simulink model "IARC_Nonlinear_Sensors"  (R2018a)
settings: Solver=ode1  StartTime=0.0  StopTime=20  FixedStep=T  RelTol=1e-3  EnableMultiTasking=on
undefined symbols (not defined in the file): A_1df, A_2df, alpha3, alpha_rp, alpha_x, alpha_z, an1, an1_v, an2, an3, bn1, bn1_v, bn2, bn3, dc_M_x, delta3, Epsilon3, F, g, Gamma1, Gamma2, Gamma3, Gamma4, gamma4_0, gamma_d_x, gamma_rp_0, gamma_x_0, gamma_z_0, Gammax, I, I_add, I_add_time, Jx, Jy, Jyaw, K, k1, k10, k11, k12, k2, k3, k4, k5, k6, k7, k8, k9, Ky, L, Light, LIMIT_CMD_PITCH, LIMIT_CMD_ROLL, LIMIT_CMD_xy, LIMIT_uCMD_HEIGHT, m, m_add, m_add_time, magnitude, MIL ... (+67)
libraries: simulink x131, simulink_extras x5, UAV_Control x4, aerolibwind2 x1
(part 2 of 6)

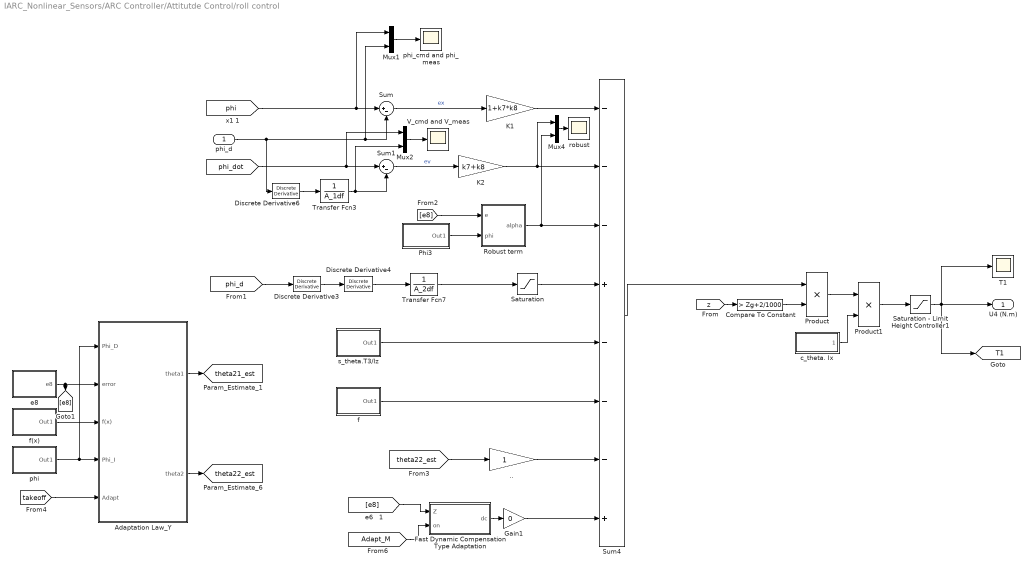
== system IARC_Nonlinear_Sensors/ARC Controller/Attitutde Control/roll control ==
  phi_d : Inport
  .. : Gain
  Adaptation Law_Y : Subsystem
  Compare To Constant : simulink/Logic and Bit Operations/Compare To Constant  relop=>  const=Zg+2/1000  OutDataTypeStr=uint8  ZeroCross=off
  Discrete Derivative3 : simulink/Discrete/Discrete Derivative  gainval=1.0  ICPrevScaledInput=0.0  OutMin=[]  OutMax=[]  OutDataType=fixdt(1, 16)  OutScaling=2^-10  DoSatur=off
  Discrete Derivative4 : simulink/Discrete/Discrete Derivative  gainval=1.0  ICPrevScaledInput=0.0  OutMin=[]  OutMax=[]  OutDataType=fixdt(1, 16)  OutScaling=2^-10  DoSatur=off
  Discrete Derivative6 : simulink/Discrete/Discrete Derivative  gainval=1.0  ICPrevScaledInput=0.0  OutMin=[]  OutMax=[]  OutDataType=fixdt(1, 16)  OutScaling=2^-10  DoSatur=off
  Fast Dynamic Compensation Type Adaptation : Subsystem  mask{dc_M=dc_M_x, gamma_d=gamma_d_x}
      mask prompts: dc_M "Bound for the lumped model compensation errors"; gamma_d "Adaptation gain:"
      mask Help:
      | d ̂  ̇_c=Proj(γ_d z)=0             if      |d ̂_c |=d_cM  and d ̂_c z>0
      |                                 γ_d z      else
      | With γ_d>0 and |d ̂_c (0)|≤d_cM
      mask Display:
      | port_label('input',1,'e','texmode','on')
      | port_label('output',1,'d_c','texmode','on')
  Gain1 : Gain  Gain=0
  K1 : Gain  Gain=1+k7*k8
  K2 : Gain  Gain=k7+k8
  Mux1 : Mux  Inputs=2
  Mux2 : Mux  Inputs=2
  Mux4 : Mux  Inputs=2
  Phi3 : Subsystem
  Product : Product  Inputs=**
  Product1 : Product
  Robust term : Subsystem  mask(Robust_Block){theta_max=theta3_Max, theta_min=theta3_Min, epsilon=Epsilon3, delta=delta3}
      mask prompts: theta_max "Maximum parameters vector value:"; theta_min "Minimum parameters vector value:"; epsilon "Error bound Coefficient:"; delta "Uncertain Nonlinearities Bound:"
      mask help: Computes the nonlinear robust feedback.
      mask Help:
      | h^2=(theta_max-theta_min)^2*phi^2+delta^2
      | u = h/(4epsilon) )e/theta
      mask Display:
      | port_label('input',1,'e','texmode','on')
      | port_label('input',2,'\phi','texmode','on')
      | 
      | port_label('output',1,'u_{s2}','texmode','on')
  Saturation : Saturate  UpperLimit=[10]  LowerLimit=[-10]
  Saturation - Limit Height Controller1 : Saturate  UpperLimit=0.8  LowerLimit=-0.8
  Sum : Sum  Inputs=|+-
  Sum1 : Sum  Inputs=|+-
  Sum4 : Sum  Inputs=---+---+
  T1 : Scope
  Transfer Fcn3 : TransferFcn  Denominator=A_1df
  Transfer Fcn7 : TransferFcn  Denominator=A_2df
  V_cmd and V_meas : Scope
  c_theta. Ix : Subsystem
  e8 : Subsystem
  f : Subsystem
  f(x) : Subsystem
  phi : Subsystem
  phi_cmd and phi_meas : Scope
  robust : Scope
  s_theta.T3/Iz : Subsystem
  U4 (N.m) : Outport
  tag scope: T1=global, theta21_est=global, theta22_est=global
  wires:
  Mux1/1 -> phi_cmd and phi_meas/1
  Sum/1 -> K1/1  "ex"
  [phi] -> Mux1/1, Sum/1
  [z] -> Compare To Constant/1
  Compare To Constant/1 -> Product/2
  Sum4/1 -> Product/1
  [phi_d] -> Discrete Derivative3/1
  Discrete Derivative3/1 -> Discrete Derivative4/1
  K1/1 -> Sum4/1
  K2/1 -> Mux4/1, Sum4/2
  Discrete Derivative4/1 -> Transfer Fcn7/1
  phi/1(Out1) -> Adaptation Law_Y/1(Phi_D), Adaptation Law_Y/4(Phi_I)
  [takeoff] -> Adaptation Law_Y/5(Adapt)
  f(x)/1(Out1) -> Adaptation Law_Y/3(f(x))
  Discrete Derivative6/1 -> Transfer Fcn3/1
  [phi_dot] -> Mux2/1, Sum1/1
  Mux2/1 -> V_cmd and V_meas/1
  e8/1(e8) -> Adaptation Law_Y/2(error), [e8]
  Adaptation Law_Y/2(theta2) -> [theta22_est]
  Adaptation Law_Y/1(theta1) -> [theta21_est]
  ../1 -> Sum4/7
  Product/1 -> Product1/1
  Phi3/1(Out1) -> Robust term/2(phi)
  Sum1/1 -> K2/1  "ev"
  [e8] -> Robust term/1(e)
  Robust term/1(alpha) -> Mux4/2, Sum4/3
  Product1/1 -> Saturation - Limit Height Controller1/1
  phi_d/1 -> Discrete Derivative6/1, Mux1/2, Sum/2
  [theta22_est] -> ../1
  s_theta.T3/Iz/1(Out1) -> Sum4/5
  f/1(Out1) -> Sum4/6
  Transfer Fcn3/1 -> Sum1/2, Mux2/2
  Saturation/1 -> Sum4/4
  Transfer Fcn7/1 -> Saturation/1
  c_theta. Ix/1(" ") -> Product1/2
  Saturation - Limit Height Controller1/1 -> [T1], T1/1, U4 (N.m)/1
  Mux4/1 -> robust/1
  [e8] -> Fast Dynamic Compensation Type Adaptation/1(Z)
  Fast Dynamic Compensation Type Adaptation/1(dc) -> Gain1/1
  [Adapt_M] -> Fast Dynamic Compensation Type Adaptation/2(on)
  Gain1/1 -> Sum4/8

== system IARC_Nonlinear_Sensors/ARC Controller/Position Control/Coupling ==
  U1 : Inport
  U2 : Inport  Port=2
  U3 : Inport  Port=3
  psi_d : Inport  Port=4
  Add : Sum  Inputs=3
  Add1 : Sum  Inputs=2
  Add2 : Sum  Inputs=+-
  Divide : Product  Inputs=*/
  Divide1 : Product  Inputs=*/
  Math Function : Math  Operator=magnitude^2  SaturateOnIntegerOverflow=on
  Math Function1 : Math  Operator=magnitude^2  SaturateOnIntegerOverflow=on
  Math Function2 : Math  Operator=magnitude^2  SaturateOnIntegerOverflow=on
  Product{,1..3} (4 alike) : Product
  Sqrt : Sqrt  SaturateOnIntegerOverflow=on
  Trigonometric Function1 : Trigonometry  Operator=asin
  Trigonometric Function2 : Trigonometry  Operator=atan
  Trigonometric Function3 : Trigonometry  Operator=sincos
  Warm Up+Sat : Subsystem
  x m_hat : Subsystem
  u1 (N) : Outport
  phi_d (rad) : Outport  Port=2
  theta_d (rad) : Outport  Port=3
  wires:
  Trigonometric Function3/1 -> Product3/2, Product1/2
  Product3/1 -> Add2/1
  Add2/1 -> Divide1/1
  Math Function2/1 -> Add/1
  Math Function/1 -> Add/3
  Add/1 -> Sqrt/1
  psi_d/1 -> Trigonometric Function3/1
  Trigonometric Function3/2 -> Product2/2, Product/2
  Add1/1 -> Divide/1
  Math Function1/1 -> Add/2
  U2/1 -> Math Function1/1, Product1/1, Product2/1
  Divide/1 -> Trigonometric Function1/1
  Divide1/1 -> Trigonometric Function2/1
  U3/1 -> Math Function/1, Divide1/2
  Product1/1 -> Add1/1
  Product/1 -> Add1/2
  U1/1 -> Product/1, Product3/1, Math Function2/1
  Product2/1 -> Add2/2
  Trigonometric Function2/1 -> phi_d (rad)/1
  Trigonometric Function1/1 -> theta_d (rad)/1
  Sqrt/1 -> Divide/2, x m_hat/1(" ")
  x m_hat/1(u1_des (N)) -> Warm Up+Sat/1(In1)
  Warm Up+Sat/1(u1 (N)) -> u1 (N)/1

== system IARC_Nonlinear_Sensors/ARC Controller/Position Control/X control ==
  Adaptation Law_X : Subsystem
  Compare To Constant : simulink/Logic and Bit Operations/Compare To Constant  relop=>  const=Zg+2/1000  OutDataTypeStr=uint8  ZeroCross=off
  Constant : Constant
  Discrete Derivative3 : simulink/Discrete/Discrete Derivative  gainval=1.0  ICPrevScaledInput=0.0  OutMin=[]  OutMax=[]  OutDataType=fixdt(1, 16)  OutScaling=2^-10  DoSatur=off
  Discrete Derivative4 : simulink/Discrete/Discrete Derivative  gainval=1.0  ICPrevScaledInput=0.0  OutMin=[]  OutMax=[]  OutDataType=fixdt(1, 16)  OutScaling=2^-10  DoSatur=off
  Discrete Derivative6 : simulink/Discrete/Discrete Derivative  gainval=1.0  ICPrevScaledInput=0.0  OutMin=[]  OutMax=[]  OutDataType=fixdt(1, 16)  OutScaling=2^-10  DoSatur=off
  Fast Dynamic Compensation Type Adaptation : Subsystem  mask{dc_M=dc_M_x, gamma_d=gamma_d_x}
      mask prompts: dc_M "Bound for the lumped model compensation errors"; gamma_d "Adaptation gain:"
      mask Help:
      | d ̂  ̇_c=Proj(γ_d z)=0             if      |d ̂_c |=d_cM  and d ̂_c z>0
      |                                 γ_d z      else
      | With γ_d>0 and |d ̂_c (0)|≤d_cM
      mask Display:
      | port_label('input',1,'e','texmode','on')
      | port_label('output',1,'d_c','texmode','on')
  Gain1 : Gain  Gain=0
  K1 : Gain  Gain=1+k1*k2
  K2 : Gain  Gain=k1+k2
  Mux1 : Mux  Inputs=2
  Mux2 : Mux  Inputs=2
  Product : Product
  Saturation1 : Saturate  UpperLimit=LIMIT_CMD_xy  LowerLimit=-LIMIT_CMD_xy
  Scope4 : Scope
  Sum : Sum  Inputs=|+-
  Sum1 : Sum  Inputs=|+-
  Sum4 : Sum  Inputs=--+-+
  V_cmd and V_meas : Scope
  X_cmd and X_meas : Scope
  e2 : Subsystem
  f(x) : Subsystem
  U1 (m/s^2) : Outport
  wires:
  Mux1/1 -> X_cmd and X_meas/1
  Sum1/1 -> K2/1  "ev"
  Sum/1 -> K1/1  "ex"
  [x] -> Mux1/1, Sum/1
  [z] -> Compare To Constant/1
  Compare To Constant/1 -> Product/2
  Product/1 -> Saturation1/1, Scope4/1
  Sum4/1 -> Product/1
  [x_des] -> Discrete Derivative3/1
  Discrete Derivative3/1 -> Discrete Derivative4/1
  K1/1 -> Sum4/1
  K2/1 -> Sum4/2
  Discrete Derivative4/1 -> Sum4/3
  Constant/1 -> Adaptation Law_X/4(Phi_d), Adaptation Law_X/2(Phi_I)
  [takeoff] -> Adaptation Law_X/3(Adapt)
  Adaptation Law_X/1(theta1) -> Sum4/4
  f(x)/1(Out1) -> Adaptation Law_X/1(f(x))
  [x_des] -> Discrete Derivative6/1, Mux1/2, Sum/2
  Discrete Derivative6/1 -> Mux2/2, Sum1/2
  [x_dot] -> Mux2/1, Sum1/1
  Mux2/1 -> V_cmd and V_meas/1
  e2/1(e2) -> [e2], Adaptation Law_X/5(error)
  Saturation1/1 -> U1 (m/s^2)/1
  [e2] -> Fast Dynamic Compensation Type Adaptation/1(Z)
  Gain1/1 -> Sum4/5
  Fast Dynamic Compensation Type Adaptation/1(dc) -> Gain1/1
  [Adapt_M] -> Fast Dynamic Compensation Type Adaptation/2(on)

== system IARC_Nonlinear_Sensors/ARC Controller/Position Control/Y control ==
  Adaptation Law_Y : Subsystem
  Compare To Constant : simulink/Logic and Bit Operations/Compare To Constant  relop=>  const=Zg+2/1000  OutDataTypeStr=uint8  ZeroCross=off
  Constant : Constant
  Discrete Derivative3 : simulink/Discrete/Discrete Derivative  gainval=1.0  ICPrevScaledInput=0.0  OutMin=[]  OutMax=[]  OutDataType=fixdt(1, 16)  OutScaling=2^-10  DoSatur=off
  Discrete Derivative4 : simulink/Discrete/Discrete Derivative  gainval=1.0  ICPrevScaledInput=0.0  OutMin=[]  OutMax=[]  OutDataType=fixdt(1, 16)  OutScaling=2^-10  DoSatur=off
  Discrete Derivative6 : simulink/Discrete/Discrete Derivative  gainval=1.0  ICPrevScaledInput=0.0  OutMin=[]  OutMax=[]  OutDataType=fixdt(1, 16)  OutScaling=2^-10  DoSatur=off
  Fast Dynamic Compensation Type Adaptation : Subsystem  mask{dc_M=dc_M_x, gamma_d=gamma_d_x}
      mask prompts: dc_M "Bound for the lumped model compensation errors"; gamma_d "Adaptation gain:"
      mask Help:
      | d ̂  ̇_c=Proj(γ_d z)=0             if      |d ̂_c |=d_cM  and d ̂_c z>0
      |                                 γ_d z      else
      | With γ_d>0 and |d ̂_c (0)|≤d_cM
      mask Display:
      | port_label('input',1,'e','texmode','on')
      | port_label('output',1,'d_c','texmode','on')
  Gain1 : Gain  Gain=0
  K1 : Gain  Gain=1+k5*k6
  K2 : Gain  Gain=k5+k6
  Mux1 : Mux  Inputs=2
  Product : Product
  Saturation1 : Saturate  UpperLimit=LIMIT_CMD_xy  LowerLimit=-LIMIT_CMD_xy
  Scope4 : Scope
  Sum : Sum  Inputs=|+-
  Sum1 : Sum  Inputs=|+-
  Sum4 : Sum  Inputs=--+-+
  e2 : Subsystem
  f(x)1 : Subsystem
  y_cmd and y_meas : Scope
  U2 (m/s^2) : Outport
  wires:
  Adaptation Law_Y/1(theta1) -> Sum4/4
  Discrete Derivative4/1 -> Sum4/3
  K2/1 -> Sum4/2
  K1/1 -> Sum4/1
  Discrete Derivative3/1 -> Discrete Derivative4/1
  [y_des] -> Discrete Derivative3/1
  Sum4/1 -> Product/1
  Product/1 -> Scope4/1, Saturation1/1
  Compare To Constant/1 -> Product/2
  [z] -> Compare To Constant/1
  [y] -> Sum/1, Mux1/1
  Sum/1 -> K1/1  "ex"
  Sum1/1 -> K2/1  "ev"
  [y_des] -> Discrete Derivative6/1, Mux1/2, Sum/2
  Mux1/1 -> y_cmd and y_meas/1
  Discrete Derivative6/1 -> Sum1/2
  [y_dot] -> Sum1/1
  f(x)1/1(Out1) -> Adaptation Law_Y/1(f(x))
  e2/1(e6) -> [e6], Adaptation Law_Y/5(error)
  Constant/1 -> Adaptation Law_Y/4(Phi_d), Adaptation Law_Y/2(Phi_I)
  [takeoff] -> Adaptation Law_Y/3(Adapt)
  Saturation1/1 -> U2 (m/s^2)/1
  Fast Dynamic Compensation Type Adaptation/1(dc) -> Gain1/1
  [e6] -> Fast Dynamic Compensation Type Adaptation/1(Z)
  [Adapt_M] -> Fast Dynamic Compensation Type Adaptation/2(on)
  Gain1/1 -> Sum4/5

== system IARC_Nonlinear_Sensors/ARC Controller/Position Control/Z control ==
  ARC block : Subsystem  AncestorBlock=UAV_Control/ARC block  mask(Robust_Block){theta_max=theta3_Max, theta_min=theta3_Min, epsilon=Epsilon3, delta=delta3}
      mask prompts: theta_max "Maximum parameters vector value:"; theta_min "Minimum parameters vector value:"; epsilon "Error bound Coefficient:"; delta "Uncertain Nonlinearities Bound:"
      mask help: Computes the nonlinear robust feedback.
      mask Help:
      | h^2=(theta_max-theta_min)^2*phi^2+delta^2
      | u = h/(4epsilon) )e/theta
      mask Display:
      | port_label('input',1,'e','texmode','on')
      | port_label('input',2,'\phi','texmode','on')
      | 
      | port_label('output',1,'u_{s2}','texmode','on')
  Constant : Constant  Value=g
  Discrete Derivative3 : simulink/Discrete/Discrete Derivative  gainval=1.0  ICPrevScaledInput=0.0  OutMin=[]  OutMax=[]  OutDataType=fixdt(1, 16)  OutScaling=2^-10  DoSatur=off
  Discrete Derivative4 : simulink/Discrete/Discrete Derivative  gainval=1.0  ICPrevScaledInput=0.0  OutMin=[]  OutMax=[]  OutDataType=fixdt(1, 16)  OutScaling=2^-10  DoSatur=off
  Discrete Derivative6 : simulink/Discrete/Discrete Derivative  gainval=1.0  ICPrevScaledInput=0.0  OutMin=[]  OutMax=[]  OutDataType=fixdt(1, 16)  OutScaling=2^-10  DoSatur=off
  Estimate theta = K/m : Subsystem
  K1 : Gain  Gain=1+k9*k10
  K2 : Gain  Gain=k9+k10
  K3 : Gain  Gain=1/100
  Mux1 : Mux  Inputs=2
  Phi : Subsystem
  Phi1 : Subsystem
  Phi3 : Subsystem
  Saturation1 : Saturate  UpperLimit=10  LowerLimit=-10
  Scope4 : Scope
  Sum : Sum  Inputs=|+-
  Sum1 : Sum  Inputs=|+-
  Sum4 : Sum  Inputs=---++-
  X_cmd and X_meas : Scope
  e10 : Subsystem
  f(x) : Subsystem
  U3 (m/s^2) : Outport
  tag scope: theta31_est=global
  wires:
  Mux1/1 -> X_cmd and X_meas/1
  [z_des] -> Discrete Derivative6/1, Sum/2, Mux1/2
  Sum1/1 -> K2/1, ARC block/1(e)  "ev"
  Discrete Derivative6/1 -> Sum1/2
  Sum/1 -> K1/1  "ex"
  [z] -> Mux1/1, Sum/1
  [z_des] -> Discrete Derivative3/1
  Discrete Derivative3/1 -> Discrete Derivative4/1
  K1/1 -> Sum4/1
  K2/1 -> Sum4/2
  Discrete Derivative4/1 -> Saturation1/1
  [Adapt_M] -> Estimate theta = K/m/5(adappt)
  Constant/1 -> Sum4/5
  f(x)/1(Out1) -> Estimate theta = K/m/3(f(f))
  Estimate theta = K/m/1(theta1) -> [theta31_est]
  Estimate theta = K/m/2(theta2) -> Sum4/6
  Phi1/1(Out1) -> Estimate theta = K/m/1(Phi_d)
  e10/1(e10) -> Estimate theta = K/m/2(error)
  Phi/1(Out1) -> Estimate theta = K/m/4(Phi)
  ARC block/1(alpha) -> K3/1
  Phi3/1(Out1) -> ARC block/2(phi)
  [z_dot] -> Sum1/1
  K3/1 -> Sum4/3
  Sum4/1 -> U3 (m/s^2)/1, Scope4/1
  Saturation1/1 -> Sum4/4

== system IARC_Nonlinear_Sensors/Generate Trajectory/adjust_for_heading3/adjust_for_heading1 ==
  x_e_d : Inport
  y_e_d : Inport  Port=2
  yaw : Inport  Port=3
  Add : Sum
  Constant : Constant  Value=yaw_control_ON
  Product : Product
  Product1 : Product
  Switch : Switch  Criteria=u2 > Threshold  Threshold=0.5
  Trigonometric Function1 : Trigonometry  Operator=sincos  OutputSignalType=real
  adj : Outport
  wires:
  yaw/1 -> Trigonometric Function1/1
  Constant/1 -> Switch/2
  y_e_d/1 -> Product/1
  x_e_d/1 -> Product1/2, Switch/3
  Trigonometric Function1/2 -> Product1/1
  Trigonometric Function1/1 -> Product/2
  Product/1 -> Add/1
  Product1/1 -> Add/2
  Add/1 -> Switch/1
  Switch/1 -> adj/1

== system IARC_Nonlinear_Sensors/Generate Trajectory/adjust_for_heading3/adjust_for_heading3 ==
  x_e_d : Inport
  y_e_d : Inport  Port=2
  yaw : Inport  Port=3
  Add : Sum  Inputs=-+
  Constant1 : Constant  Value=yaw_control_ON
  Product : Product
  Product1 : Product
  Switch1 : Switch  Criteria=u2 > Threshold  Threshold=0.5
  Trigonometric Function1 : Trigonometry  Operator=sincos  OutputSignalType=real
  adj : Outport
  wires:
  yaw/1 -> Trigonometric Function1/1
  Constant1/1 -> Switch1/2
  x_e_d/1 -> Product/1
  y_e_d/1 -> Switch1/3, Product1/2
  Trigonometric Function1/2 -> Product1/1
  Trigonometric Function1/1 -> Product/2
  Product/1 -> Add/1
  Product1/1 -> Add/2
  Add/1 -> Switch1/1
  Switch1/1 -> adj/1

== system IARC_Nonlinear_Sensors/Generate Trajectory/steady takeoff (x)/Triggered Subsystem1 ==
  " " : Inport
  Trigger : TriggerPort  VariantControl=(inherit)
  "  " : Outport
  wires:
  " "/1 -> "  "/1

== system IARC_Nonlinear_Sensors/Generate Trajectory/steady takeoff (x)/Triggered Subsystem2 ==
  " " : Inport
  Trigger : TriggerPort  VariantControl=(inherit)
  "  " : Outport
  wires:
  " "/1 -> "  "/1

== system IARC_Nonlinear_Sensors/Generate Trajectory/steady takeoff (y)/Triggered Subsystem1 ==
  " " : Inport
  Trigger : TriggerPort  VariantControl=(inherit)
  "  " : Outport
  wires:
  " "/1 -> "  "/1

== system IARC_Nonlinear_Sensors/Generate Trajectory/steady takeoff (y)/Triggered Subsystem2 ==
  " " : Inport
  Trigger : TriggerPort  VariantControl=(inherit)
  "  " : Outport
  wires:
  " "/1 -> "  "/1

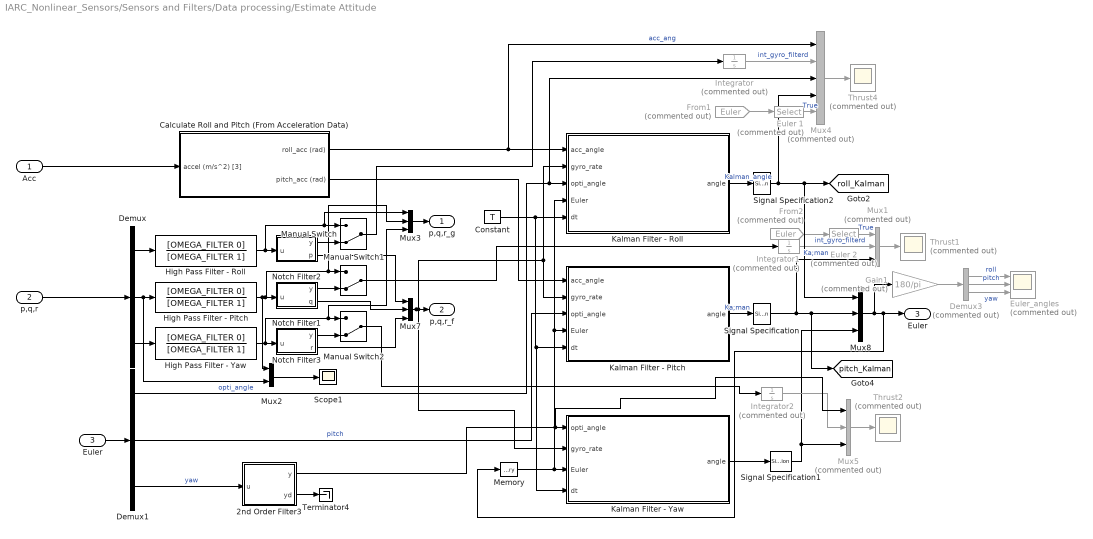
== system IARC_Nonlinear_Sensors/Sensors and Filters/Data processing/Estimate Attitude ==
  Acc : Inport
  p,q,r : Inport  Port=2
  Euler : Inport  Port=3
  2nd Order Filter3 : Subsystem
  Calculate Roll and Pitch (From Acceleration Data) : Subsystem
  Constant : Constant  Value=T
  Demux : Demux  Outputs=3
  Demux1 : Demux  Outputs=3
  Demux3 : Demux  Commented=on  Outputs=3
  Euler 1 : Selector  Commented=on  InputPortWidth=3  IndexOptions=Index vector (dialog)  Indices=1  OutputSizes=1
  Euler 2 : Selector  Commented=on  InputPortWidth=3  IndexOptions=Index vector (dialog)  Indices=2  OutputSizes=1
  Euler_angles : Scope  Commented=on  NumInputPorts=3
  From1 : From  Commented=on  GotoTag=Euler  TagVisibility=global
  From2 : From  Commented=on  GotoTag=Euler  TagVisibility=global
  Gain1 : Gain  Commented=on  Gain=180/pi
  High Pass Filter - Pitch : TransferFcn  Numerator=[OMEGA_FILTER 0]  Denominator=[OMEGA_FILTER 1]
  High Pass Filter - Roll : TransferFcn  Numerator=[OMEGA_FILTER 0]  Denominator=[OMEGA_FILTER 1]
  High Pass Filter - Yaw : TransferFcn  Numerator=[OMEGA_FILTER 0]  Denominator=[OMEGA_FILTER 1]
  Integrator : Integrator  Commented=on
  Integrator1 : Integrator  Commented=on
  Integrator2 : Integrator  Commented=on
  Kalman Filter - Pitch : MATLAB Function  TreatAsAtomicUnit=on
  Kalman Filter - Roll : MATLAB Function  TreatAsAtomicUnit=on
  Kalman Filter - Yaw : MATLAB Function  TreatAsAtomicUnit=on
  Manual Switch : ManualSwitch  CurrentSetting=0
  Manual Switch1 : ManualSwitch  CurrentSetting=0
  Manual Switch2 : ManualSwitch  CurrentSetting=0
  Memory : Memory
  Mux1 : Mux  Commented=on  Inputs=3
  Mux2 : Mux  Inputs=2
  Mux3 : Mux  Inputs=3
  Mux4 : Mux  Commented=on  Inputs=5
  Mux5 : Mux  Commented=on  Inputs=3
  Mux7 : Mux  Inputs=3
  Mux8 : Mux  Inputs=3
  Notch Filter1 : Subsystem
  Notch Filter2 : Subsystem
  Notch Filter3 : Subsystem
  Scope1 : Scope
  Signal Specification : SignalSpecification  Dimensions=1
  Signal Specification1 : SignalSpecification  Dimensions=1
  Signal Specification2 : SignalSpecification  Dimensions=1
  Terminator4 : Terminator
  Thrust1 : Scope  Commented=on
  Thrust2 : Scope  Commented=on
  Thrust4 : Scope  Commented=on
  p,q,r_g : Outport
  p,q,r_f : Outport  Port=2
  " Euler" : Outport  Port=3
  tag scope: pitch_Kalman=global, roll_Kalman=global
  wires:
  Demux1/1 -> Mux4/3, Kalman Filter - Roll/3(opti_angle)  "opti_angle"
  Demux/2 -> Mux2/2, High Pass Filter - Pitch/1
  Mux7/1 -> Kalman Filter - Roll/2(gyro_rate), Kalman Filter - Pitch/2(gyro_rate), Kalman Filter - Yaw/2(gyro_rate), p,q,r_f/1
  Manual Switch2/1 -> Integrator2/1
  Calculate Roll and Pitch (From Acceleration Data)/2(pitch_acc (rad)) -> Kalman Filter - Pitch/1(acc_angle)
  Gain1/1 -> Demux3/1
  Kalman Filter - Roll/1(angle) -> Signal Specification2/1  "Kalman_angle"
  Demux/3 -> High Pass Filter - Yaw/1
  Demux1/3 -> 2nd Order Filter3/1(u)  "yaw"
  p,q,r/1 -> Demux/1
  2nd Order Filter3/2(yd) -> Terminator4/1
  Demux/1 -> High Pass Filter - Roll/1
  Mux4/1 -> Thrust4/1
  Manual Switch/1 -> Integrator/1
  Mux8/1 -> Memory/1, " Euler"/1, Gain1/1
  Manual Switch1/1 -> Integrator1/1
  Integrator/1 -> Mux4/2  "int_gyro_filterd"
  Euler 1/1 -> Mux4/5  "True"
  Signal Specification/1 -> [pitch_Kalman], Mux8/2, Mux1/3  "Ka;man"
  Calculate Roll and Pitch (From Acceleration Data)/1(roll_acc (rad)) -> Mux4/1, Kalman Filter - Roll/1(acc_angle)  "acc_ang"
  Demux1/2 -> Kalman Filter - Pitch/3(opti_angle)  "pitch"
  Demux3/3 -> Euler_angles/3  "yaw"
  From1/1 -> Euler 1/1
  Constant/1 -> Kalman Filter - Yaw/4(dt), Kalman Filter - Pitch/5(dt), Kalman Filter - Roll/5(dt)
  Demux3/2 -> Euler_angles/2  "pitch"
  Demux3/1 -> Euler_angles/1  "roll"
  Euler/1 -> Demux1/1
  Acc/1 -> Calculate Roll and Pitch (From Acceleration Data)/1(accel (m/s^2) [3])
  High Pass Filter - Roll/1 -> Notch Filter2/1(u), Mux3/1, Manual Switch/1
  Notch Filter2/1(y) -> Manual Switch/2
  Notch Filter1/1(y) -> Manual Switch1/2
  High Pass Filter - Pitch/1 -> Mux2/1, Mux3/2, Manual Switch1/1, Notch Filter1/1(u)
  High Pass Filter - Yaw/1 -> Notch Filter3/1(u), Mux3/3, Manual Switch2/1
  Notch Filter3/1(y) -> Manual Switch2/2
  Mux1/1 -> Thrust1/1
  Integrator1/1 -> Mux1/2  "int_gyro_filterd"
  From2/1 -> Euler 2/1
  Euler 2/1 -> Mux1/1  "True"
  Mux2/1 -> Scope1/1
  Mux3/1 -> p,q,r_g/1
  Mux5/1 -> Thrust2/1
  Signal Specification1/1 -> Mux5/3, Mux8/3
  Integrator2/1 -> Mux5/2
  Notch Filter2/2(p) -> Mux7/1
  Notch Filter1/2(q) -> Mux7/2
  Notch Filter3/2(r) -> Mux7/3
  Memory/1 -> Kalman Filter - Yaw/3(Euler), Kalman Filter - Roll/4(Euler), Kalman Filter - Pitch/4(Euler)
  2nd Order Filter3/1(y) -> Mux5/1, Kalman Filter - Yaw/1(opti_angle)
  Kalman Filter - Yaw/1(angle) -> Signal Specification1/1
  Kalman Filter - Pitch/1(angle) -> Signal Specification/1  "Ka;man"
  Signal Specification2/1 -> Mux8/1, [roll_Kalman], Mux4/4

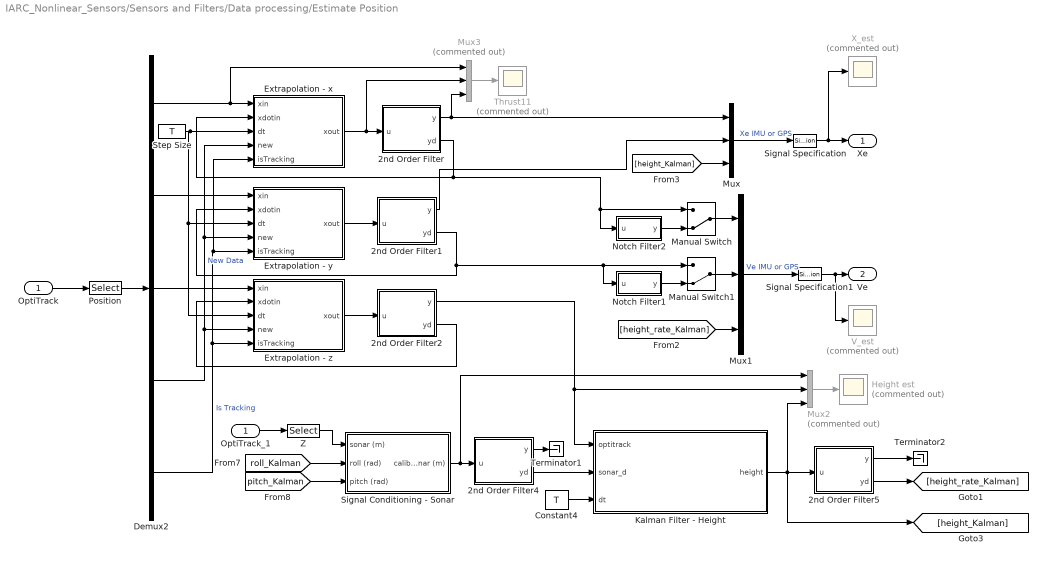
== system IARC_Nonlinear_Sensors/Sensors and Filters/Data processing/Estimate Position ==
  OptiTrack : Inport
  2nd Order Filter : Subsystem
  2nd Order Filter1 : Subsystem
  2nd Order Filter2 : Subsystem
  2nd Order Filter4 : Subsystem
  2nd Order Filter5 : Subsystem
  Constant4 : Constant  Value=T
  Demux2 : Demux  Outputs=5
  Extrapolation - x : MATLAB Function  TreatAsAtomicUnit=on
  Extrapolation - y : MATLAB Function  TreatAsAtomicUnit=on
  Extrapolation - z : MATLAB Function  TreatAsAtomicUnit=on
  Height est : Scope  Commented=on
  Kalman Filter - Height : MATLAB Function  TreatAsAtomicUnit=on
  Manual Switch : ManualSwitch  CurrentSetting=0
  Manual Switch1 : ManualSwitch  CurrentSetting=0
  Mux : Mux  Inputs=3
  Mux1 : Mux  Inputs=3
  Mux2 : Mux  Commented=on  Inputs=3
  Mux3 : Mux  Commented=on  Inputs=3
  Notch Filter1 : Subsystem
  Notch Filter2 : Subsystem
  OptiTrack_1 : InportShadow
  Position : Selector  InputPortWidth=8  IndexOptions=Index vector (dialog)  Indices=[1 2 3 7 8]  OutputSizes=1
  Signal Conditioning - Sonar : Subsystem
  Signal Specification : SignalSpecification  Dimensions=3
  Signal Specification1 : SignalSpecification  Dimensions=3
  Step Size : Constant  Value=T
  Terminator1 : Terminator
  Terminator2 : Terminator
  Thrust11 : Scope  Commented=on
  V_est : Scope  Commented=on
  X_est : Scope  Commented=on
  Z : Selector  InputPortWidth=8  IndexOptions=Index vector (dialog)  Indices=[3]  OutputSizes=1
  Xe : Outport
  Ve : Outport  Port=2
  wires:
  Demux2/1 -> Mux3/1, Extrapolation - x/1(xin)
  2nd Order Filter5/2(yd) -> [height_rate_Kalman]
  Demux2/4 -> Extrapolation - z/4(new), Extrapolation - y/4(new), Extrapolation - x/4(new)  "New Data"
  Constant4/1 -> Kalman Filter - Height/3(dt)
  2nd Order Filter1/2(yd) -> Extrapolation - y/2(xdotin), Notch Filter1/1(u), Manual Switch1/1
  Extrapolation - x/1(xout) -> Mux3/2, 2nd Order Filter/1(u)
  2nd Order Filter/1(y) -> Mux3/3, Mux/1
  Extrapolation - z/1(xout) -> 2nd Order Filter2/1(u)
  2nd Order Filter4/2(yd) -> Kalman Filter - Height/2(sonar_d)
  Z/1 -> Signal Conditioning - Sonar/1(sonar (m))
  2nd Order Filter2/1(y) -> Kalman Filter - Height/1(optitrack), Mux2/2
  [pitch_Kalman] -> Signal Conditioning - Sonar/3(pitch (rad))
  Kalman Filter - Height/1(height) -> Mux2/3, [height_Kalman], 2nd Order Filter5/1(u)
  OptiTrack_1/1 -> Z/1
  2nd Order Filter4/1(y) -> Terminator1/1
  Signal Conditioning - Sonar/1(calib sonar (m)) -> Mux2/1, 2nd Order Filter4/1(u)
  Step Size/1 -> Extrapolation - z/3(dt), Extrapolation - y/3(dt), Extrapolation - x/3(dt)
  Position/1 -> Demux2/1
  Demux2/3 -> Extrapolation - z/1(xin)
  [roll_Kalman] -> Signal Conditioning - Sonar/2(roll (rad))
  2nd Order Filter5/1(y) -> Terminator2/1
  Mux/1 -> Signal Specification/1  "Xe IMU or GPS"
  [height_rate_Kalman] -> Mux1/3
  Demux2/5 -> Extrapolation - x/5(isTracking), Extrapolation - y/5(isTracking), Extrapolation - z/5(isTracking)  "Is Tracking"
  Mux2/1 -> Height est/1
  Mux1/1 -> Signal Specification1/1  "Ve IMU or GPS"
  Demux2/2 -> Extrapolation - y/1(xin)
  OptiTrack/1 -> Position/1
  Mux3/1 -> Thrust11/1
  Extrapolation - y/1(xout) -> 2nd Order Filter1/1(u)
  2nd Order Filter2/2(yd) -> Extrapolation - z/2(xdotin)
  2nd Order Filter1/1(y) -> Mux/2
  [height_Kalman] -> Mux/3
  Notch Filter2/1(y) -> Manual Switch/2
  2nd Order Filter/2(yd) -> Notch Filter2/1(u), Manual Switch/1, Extrapolation - x/2(xdotin)
  Manual Switch/1 -> Mux1/1
  Manual Switch1/1 -> Mux1/2
  Notch Filter1/1(y) -> Manual Switch1/2
  Signal Specification/1 -> Xe/1, X_est/1
  Signal Specification1/1 -> Ve/1, V_est/1

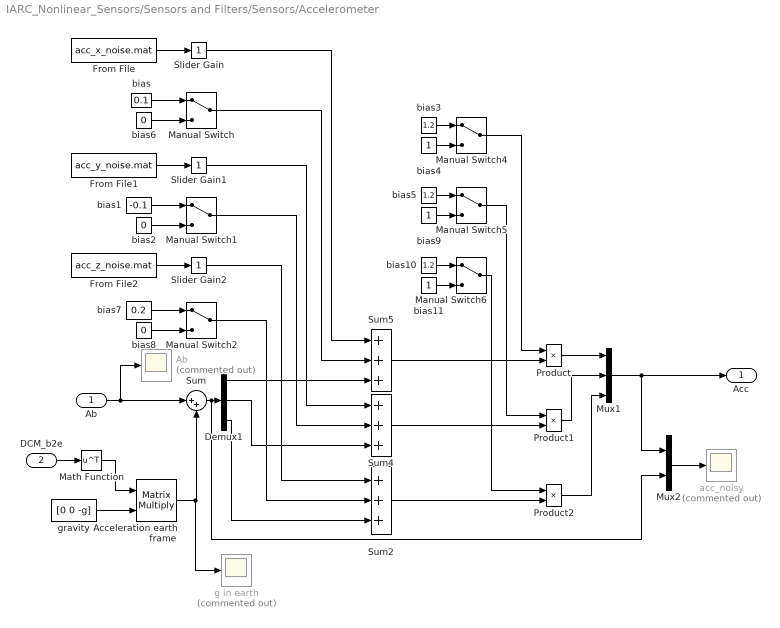
== system IARC_Nonlinear_Sensors/Sensors and Filters/Sensors/Accelerometer ==
  Ab : Inport
  DCM_b2e : Inport  Port=2
  "Ab " : Scope  Commented=on
  Acceleration earth frame : Product  Multiplication=Matrix(*)
  Demux1 : Demux  Outputs=3
  From File : FromFile  FileName=acc_x_noise.mat  SampleTime=0
  From File1 : FromFile  FileName=acc_y_noise.mat  SampleTime=0
  From File2 : FromFile  FileName=acc_z_noise.mat  SampleTime=0
  Manual Switch{,1..2,4..6} (6 alike) : ManualSwitch
  Math Function : Math  Operator=transpose  SaturateOnIntegerOverflow=on
  Mux1 : Mux  Inputs=3
  Mux2 : Mux  Inputs=2
  Product : Product  SaturateOnIntegerOverflow=on  RndMeth=Zero  InputSameDT=on  OutDataTypeStr=Inherit: Same as first input
  Product1 : Product  SaturateOnIntegerOverflow=on  RndMeth=Zero  InputSameDT=on  OutDataTypeStr=Inherit: Same as first input
  Product2 : Product  SaturateOnIntegerOverflow=on  RndMeth=Zero  InputSameDT=on  OutDataTypeStr=Inherit: Same as first input
  Slider Gain : simulink/Math Operations/Slider Gain  gain=1  low=0  high=2
  Slider Gain1 : simulink/Math Operations/Slider Gain  gain=1  low=0  high=2
  Slider Gain2 : simulink/Math Operations/Slider Gain  gain=1  low=0  high=2
  Sum : Sum  Inputs=|++
  Sum2 : Sum  Inputs=+++  SaturateOnIntegerOverflow=on  InputSameDT=on  OutDataTypeStr=Inherit: Same as first input
  Sum4 : Sum  Inputs=+++  SaturateOnIntegerOverflow=on  InputSameDT=on  OutDataTypeStr=Inherit: Same as first input
  Sum5 : Sum  Inputs=+++  SaturateOnIntegerOverflow=on  InputSameDT=on  OutDataTypeStr=Inherit: Same as first input
  acc_noisy : Scope  Commented=on
  bias : Constant  Value=0.1  VectorParams1D=off
  bias1 : Constant  Value=-0.1  VectorParams1D=off
  bias10 : Constant  Value=1.2  VectorParams1D=off
  bias11 : Constant  VectorParams1D=off
  bias2 : Constant  Value=0  VectorParams1D=off
  bias3 : Constant  Value=1.2  VectorParams1D=off
  bias4 : Constant  VectorParams1D=off
  bias5 : Constant  Value=1.2  VectorParams1D=off
  bias6 : Constant  Value=0  VectorParams1D=off
  bias7 : Constant  Value=0.2  VectorParams1D=off
  bias8 : Constant  Value=0  VectorParams1D=off
  bias9 : Constant  VectorParams1D=off
  g in earth : Scope  Commented=on
  gravity : Constant  Value=[0 0 -g]
  Acc : Outport
  wires:
  bias11/1 -> Manual Switch6/2
  bias10/1 -> Manual Switch6/1
  bias9/1 -> Manual Switch5/2
  bias5/1 -> Manual Switch5/1
  bias4/1 -> Manual Switch4/2
  bias3/1 -> Manual Switch4/1
  Manual Switch1/1 -> Sum4/2
  Manual Switch2/1 -> Sum2/2
  bias8/1 -> Manual Switch2/2
  bias7/1 -> Manual Switch2/1
  bias2/1 -> Manual Switch1/2
  bias1/1 -> Manual Switch1/1
  bias6/1 -> Manual Switch/2
  bias/1 -> Manual Switch/1
  Manual Switch/1 -> Sum5/2
  Manual Switch5/1 -> Product1/1
  Manual Switch6/1 -> Product2/1
  Manual Switch4/1 -> Product/1
  Product2/1 -> Mux1/3
  Sum2/1 -> Product2/2
  Product1/1 -> Mux1/2
  Sum4/1 -> Product1/2
  Product/1 -> Mux1/1
  Sum5/1 -> Product/2
  Slider Gain/1 -> Sum5/1
  Slider Gain1/1 -> Sum4/1
  Slider Gain2/1 -> Sum2/1
  From File2/1 -> Slider Gain2/1
  From File1/1 -> Slider Gain1/1
  Demux1/1 -> Sum5/3
  Demux1/2 -> Sum4/3
  Demux1/3 -> Sum2/3
  From File/1 -> Slider Gain/1
  gravity/1 -> Acceleration earth frame/2
  DCM_b2e/1 -> Math Function/1
  Acceleration earth frame/1 -> g in earth/1, Sum/2
  Ab/1 -> "Ab "/1, Sum/1
  Math Function/1 -> Acceleration earth frame/1
  Mux2/1 -> acc_noisy/1
  Mux1/1 -> Mux2/1, Acc/1
  Sum/1 -> Mux2/2, Demux1/1

== system IARC_Nonlinear_Sensors/Sensors and Filters/Sensors/Gyro ==
  note: 0.25
  note: 1
  p,q,r : Inport
  Degrees to Radians2 : simulink_extras/Transformations/Degrees to Radians
  Degrees to Radians3 : simulink_extras/Transformations/Degrees to Radians
  Degrees to Radians4 : simulink_extras/Transformations/Degrees to Radians
  Demux3 : Demux  Outputs=3
  From File : FromFile  FileName=gyro_p_noise.mat  SampleTime=0
  From File1 : FromFile  FileName=gyro_q_noise.mat  SampleTime=0
  From File2 : FromFile  FileName=gyro_r_noise.mat  SampleTime=0
  Manual Switch : ManualSwitch
  Manual Switch1 : ManualSwitch
  Manual Switch2 : ManualSwitch
  Manual Switch4 : ManualSwitch  CurrentSetting=0
  Manual Switch5 : ManualSwitch  CurrentSetting=0
  Manual Switch6 : ManualSwitch  CurrentSetting=0
  Mux1 : Mux  Inputs=3
  Product : Product  SaturateOnIntegerOverflow=on  RndMeth=Zero  InputSameDT=on  OutDataTypeStr=Inherit: Same as first input
  Product1 : Product  SaturateOnIntegerOverflow=on  RndMeth=Zero  InputSameDT=on  OutDataTypeStr=Inherit: Same as first input
  Product2 : Product  SaturateOnIntegerOverflow=on  RndMeth=Zero  InputSameDT=on  OutDataTypeStr=Inherit: Same as first input
  Slider Gain : simulink/Math Operations/Slider Gain  gain=1  low=0  high=2
  Slider Gain1 : simulink/Math Operations/Slider Gain  gain=1  low=0  high=2
  Slider Gain2 : simulink/Math Operations/Slider Gain  gain=0.5  low=0  high=2
  Sum1 : Sum  Inputs=+++  SaturateOnIntegerOverflow=on  InputSameDT=on  OutDataTypeStr=Inherit: Same as first input
  Sum2 : Sum  Inputs=+++  SaturateOnIntegerOverflow=on  InputSameDT=on  OutDataTypeStr=Inherit: Same as first input
  Sum3 : Sum  Inputs=+++  SaturateOnIntegerOverflow=on  InputSameDT=on  OutDataTypeStr=Inherit: Same as first input
  Variable Integer Delay3 : Delay  DelayLength=0
  bias{,4,7,9,11} (5 alike) : Constant  VectorParams1D=off
  bias1 : Constant  Value=-1  VectorParams1D=off
  bias10 : Constant  Value=0.9  VectorParams1D=off
  bias2 : Constant  Value=0  VectorParams1D=off
  bias3 : Constant  Value=0.9  VectorParams1D=off
  bias5 : Constant  Value=0.9  VectorParams1D=off
  bias6 : Constant  Value=0  VectorParams1D=off
  bias8 : Constant  Value=0  VectorParams1D=off
  "p,q,r " : Outport
  wires:
  bias11/1 -> Manual Switch6/2
  bias10/1 -> Manual Switch6/1
  bias9/1 -> Manual Switch5/2
  bias5/1 -> Manual Switch5/1
  bias4/1 -> Manual Switch4/2
  bias3/1 -> Manual Switch4/1
  Manual Switch1/1 -> Degrees to Radians2/1
  Manual Switch2/1 -> Degrees to Radians4/1
  bias8/1 -> Manual Switch2/2
  bias7/1 -> Manual Switch2/1
  bias2/1 -> Manual Switch1/2
  bias1/1 -> Manual Switch1/1
  bias6/1 -> Manual Switch/2
  bias/1 -> Manual Switch/1
  Manual Switch/1 -> Degrees to Radians3/1
  Degrees to Radians4/1 -> Sum1/2
  Degrees to Radians2/1 -> Sum2/2
  Degrees to Radians3/1 -> Sum3/2
  Manual Switch5/1 -> Product1/1
  Manual Switch6/1 -> Product2/1
  Manual Switch4/1 -> Product/1
  Product2/1 -> Mux1/3
  Sum1/1 -> Product2/2
  Product1/1 -> Mux1/2
  Sum2/1 -> Product1/2
  Product/1 -> Mux1/1
  Slider Gain/1 -> Sum3/1
  Slider Gain1/1 -> Sum2/1
  Slider Gain2/1 -> Sum1/1
  From File2/1 -> Slider Gain2/1
  From File1/1 -> Slider Gain1/1
  Demux3/1 -> Sum3/3
  Demux3/2 -> Sum2/3
  Demux3/3 -> Sum1/3
  From File/1 -> Slider Gain/1
  p,q,r/1 -> Demux3/1
  Mux1/1 -> Variable Integer Delay3/1
  Sum3/1 -> Product/2
  Variable Integer Delay3/1 -> "p,q,r "/1

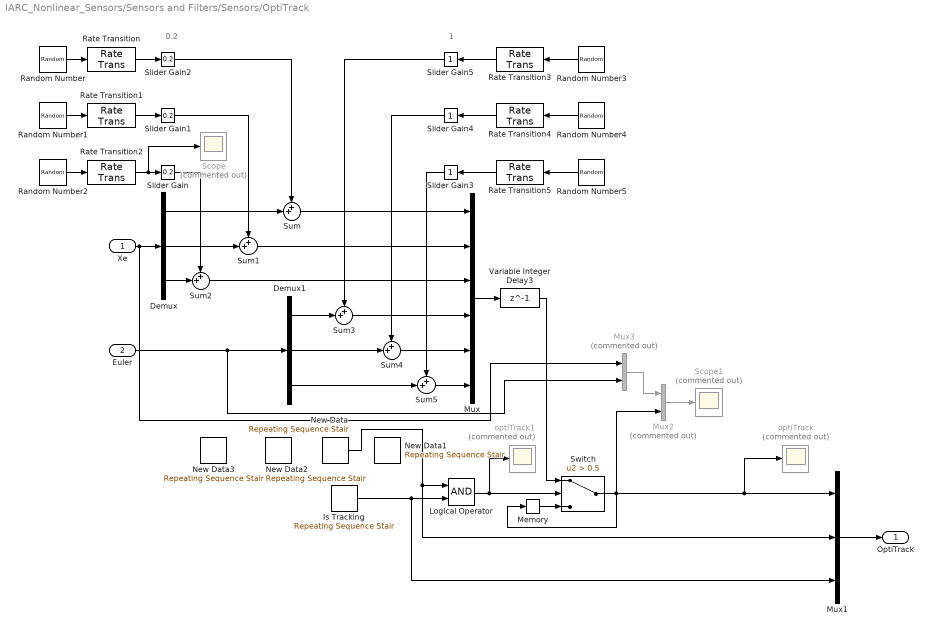
== system IARC_Nonlinear_Sensors/Sensors and Filters/Sensors/OptiTrack  ==
  note: 0.2
  note: 1
  Xe : Inport
  Euler : Inport  Port=2
  Demux : Demux  Outputs=3
  Demux1 : Demux  Outputs=3
  Is Tracking : simulink/Sources/Repeating Sequence Stair  OutValues=[1 1 1 1 1 1 1 1 1 1 1 1 1 1 1 1 1 1 1 1]  tsamp=-1  OutMin=[]  OutMax=[]  OutDataTypeStr=double  OutputDataTypeScalingMode=double  OutDataType=fixdt(0,8)  ConRadixGroup=Best Precision: Vector-wise  OutScaling=2^-12
  Logical Operator : Logic  AllPortsSameDT=off  OutDataTypeStr=boolean
  Memory : Memory
  Mux : Mux  Inputs=6
  Mux1 : Mux  Inputs=3
  Mux2 : Mux  Commented=on  Inputs=2
  Mux3 : Mux  Commented=on  Inputs=2
  New Data : simulink/Sources/Repeating Sequence Stair  OutValues=[1 1 1 0 0 1 0 1 1 1 1 0 1 1 0 1 1 1 1 1 0 0 0 1 1 0 1 1 1 0]  tsamp=-1  OutMin=[]  OutMax=[]  OutDataTypeStr=double  OutputDataTypeScalingMode=double  OutDataType=fixdt(0,8)  ConRadixGroup=Best Precision: Vector-wise  OutScaling=2^-12
  New Data1 : simulink/Sources/Repeating Sequence Stair  OutValues=[1 1 1]  tsamp=-1  OutMin=[]  OutMax=[]  OutDataTypeStr=double  OutputDataTypeScalingMode=double  OutDataType=fixdt(0,8)  ConRadixGroup=Best Precision: Vector-wise  OutScaling=2^-12
  New Data2 : simulink/Sources/Repeating Sequence Stair  OutValues=[1 0 1 0 1 0 1 0 0 1 0 0 1 0 1 0 1 0 0 0 1 0 0 0 1 0 1 0 1 0 1 0 1 0 0 1 0 0]  tsamp=-1  OutMin=[]  OutMax=[]  OutDataTypeStr=double  OutputDataTypeScalingMode=double  OutDataType=fixdt(0,8)  ConRadixGroup=Best Precision: Vector-wise  OutScaling=2^-12
  New Data3 : simulink/Sources/Repeating Sequence Stair  OutValues=[1 1 1 1 1 1 1 1 1 1 1 1 1 1 1 1 1 1 1 1 1 1 1 1 0 0 0 1 0 0 1 0 1]  tsamp=-1  OutMin=[]  OutMax=[]  OutDataTypeStr=double  OutputDataTypeScalingMode=double  OutDataType=fixdt(0,8)  ConRadixGroup=Best Precision: Vector-wise  OutScaling=2^-12
  Random Number : RandomNumber  Variance=1/1000000  SampleTime=T*3
  Random Number1 : RandomNumber  Variance=1/1000000  SampleTime=T*3
  Random Number2 : RandomNumber  Variance=1/1000000  SampleTime=T*3
  Random Number3 : RandomNumber  Variance=1/10000000  SampleTime=T*3
  Random Number4 : RandomNumber  Variance=1/10000000  SampleTime=T*3
  Random Number5 : RandomNumber  Variance=1/10000000  SampleTime=T*3
  Rate Transition{,1..5} (6 alike) : RateTransition
  Scope : Scope  Commented=on
  Scope1 : Scope  Commented=on
  Slider Gain : simulink/Math Operations/Slider Gain  gain=0.2  low=0  high=2
  Slider Gain1 : simulink/Math Operations/Slider Gain  gain=0.2  low=0  high=2
  Slider Gain2 : simulink/Math Operations/Slider Gain  gain=0.2  low=0  high=2
  Slider Gain3 : simulink/Math Operations/Slider Gain  gain=1  low=0  high=2
  Slider Gain4 : simulink/Math Operations/Slider Gain  gain=1  low=0  high=2
  Slider Gain5 : simulink/Math Operations/Slider Gain  gain=1  low=0  high=2
  Sum{,1..5} (6 alike) : Sum  Inputs=++|
  Switch : Switch  Criteria=u2 > Threshold  Threshold=0.5
  Variable Integer Delay3 : Delay  DelayLength=1
  optiTrack : Scope  Commented=on
  optiTrack1 : Scope  Commented=on
  OptiTrack : Outport
  wires:
  Mux/1 -> Variable Integer Delay3/1
  New Data/1 -> Mux1/2, Logical Operator/1
  Is Tracking/1 -> Mux1/3, Logical Operator/2
  Logical Operator/1 -> optiTrack1/1, Switch/2
  Memory/1 -> Switch/3
  Slider Gain/1 -> Sum2/1
  Random Number2/1 -> Rate Transition2/1
  Xe/1 -> Mux3/1, Demux/1
  Demux/1 -> Sum/2
  Demux/2 -> Sum1/2
  Demux/3 -> Sum2/2
  Sum2/1 -> Mux/3
  Sum1/1 -> Mux/2
  Sum/1 -> Mux/1
  Random Number1/1 -> Rate Transition1/1
  Random Number/1 -> Rate Transition/1
  Slider Gain1/1 -> Sum1/1
  Slider Gain2/1 -> Sum/1
  Mux1/1 -> OptiTrack/1
  Mux2/1 -> Scope1/1
  Euler/1 -> Mux3/2, Demux1/1
  Random Number3/1 -> Rate Transition3/1
  Random Number4/1 -> Rate Transition4/1
  Random Number5/1 -> Rate Transition5/1
  Demux1/1 -> Sum3/2
  Demux1/2 -> Sum4/2
  Sum4/1 -> Mux/5
  Demux1/3 -> Sum5/2
  Sum5/1 -> Mux/6
  Slider Gain5/1 -> Sum3/1
  Slider Gain4/1 -> Sum4/1
  Sum3/1 -> Mux/4
  Slider Gain3/1 -> Sum5/1
  Variable Integer Delay3/1 -> Switch/1
  Rate Transition/1 -> Slider Gain2/1
  Rate Transition1/1 -> Slider Gain1/1
  Rate Transition2/1 -> Scope/1, Slider Gain/1
  Rate Transition3/1 -> Slider Gain5/1
  Rate Transition4/1 -> Slider Gain4/1
  Rate Transition5/1 -> Slider Gain3/1
  Mux3/1 -> Mux2/1
  Switch/1 -> optiTrack/1, Mux1/1, Mux2/2, Memory/1

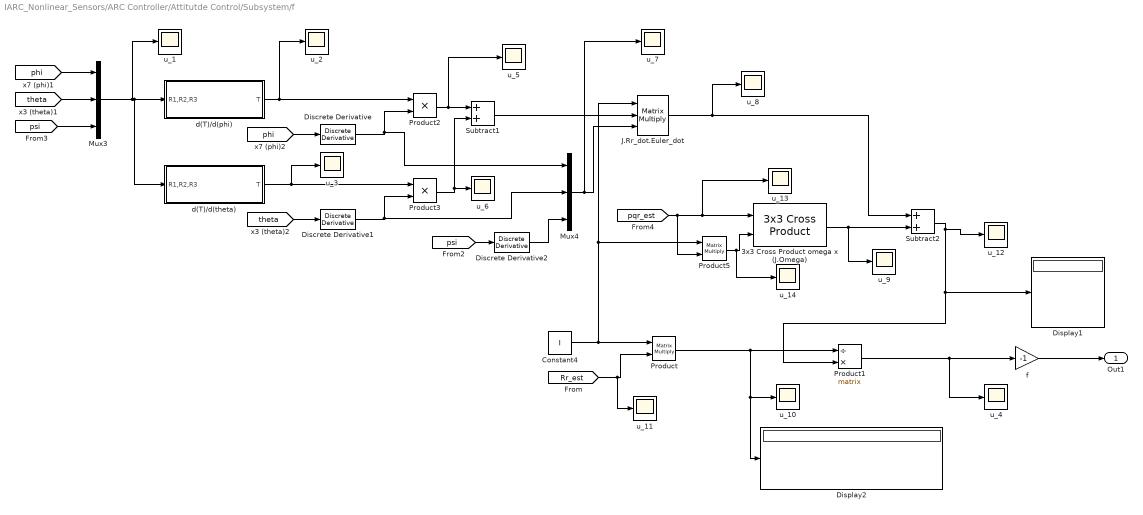
== system IARC_Nonlinear_Sensors/ARC Controller/Attitutde Control/Subsystem/f ==
  3x3 Cross Product omega x (J.Omega) : UAV_Control/3x3 Cross Product
      settings: SourceProductName=UAV_Control
  Constant4 : Constant  Value=I
  Discrete Derivative : simulink/Discrete/Discrete Derivative  gainval=1.0  ICPrevScaledInput=0.0  OutMin=[]  OutMax=[]  OutDataType=fixdt(1, 16)  OutScaling=2^-10  DoSatur=off
  Discrete Derivative1 : simulink/Discrete/Discrete Derivative  gainval=1.0  ICPrevScaledInput=0.0  OutMin=[]  OutMax=[]  OutDataType=fixdt(1, 16)  OutScaling=2^-10  DoSatur=off
  Discrete Derivative2 : simulink/Discrete/Discrete Derivative  gainval=1.0  ICPrevScaledInput=0.0  OutMin=[]  OutMax=[]  OutDataType=fixdt(1, 16)  OutScaling=2^-10  DoSatur=off
  Display1 : Display
  Display2 : Display
  J.Rr_dot.Euler_dot : Product  Inputs=3  Multiplication=Matrix(*)
  Mux3 : Mux  Inputs=3
  Mux4 : Mux  Inputs=3
  Product : Product  Multiplication=Matrix(*)
  Product1 : Product  Inputs=/*  Multiplication=Matrix(*)
  Product2 : Product
  Product3 : Product
  Product5 : Product  Multiplication=Matrix(*)
  Subtract1 : Sum
  Subtract2 : Sum
  d(T)/d(phi) : Subsystem
      mask help: d(T)/d(phi)
      mask Display:
      | port_label('input',1,'[R_1,R_2,R_3]','texmode','on')
      | port_label('output',1,'T_{eb}','texmode','on')
  d(T)/d(theta) : Subsystem
      mask help: d(T)/d(phi)
      mask Display:
      | port_label('input',1,'[R_1,R_2,R_3]','texmode','on')
      | port_label('output',1,'T_{eb}','texmode','on')
  f : Gain  Gain=-1
  u_{1..14} (14 alike) : Scope
  Out1 : Outport
  wires:
  3x3 Cross Product omega x (J.Omega)/1 -> u_9/1, Subtract2/2
  Product5/1 -> u_14/1, 3x3 Cross Product omega x (J.Omega)/2
  [pqr_est] -> Product5/2, u_13/1, 3x3 Cross Product omega x (J.Omega)/1
  [theta] -> Mux3/2
  d(T)/d(phi)/1(T) -> u_2/1, Product2/1
  Constant4/1 -> Product/1, J.Rr_dot.Euler_dot/1, Product5/1
  [theta] -> Discrete Derivative1/1
  Mux3/1 -> u_1/1, d(T)/d(theta)/1(R1,R2,R3), d(T)/d(phi)/1(R1,R2,R3)
  Discrete Derivative/1 -> Mux4/1, Product2/2
  [Rr_est] -> u_11/1, Product/2
  [phi] -> Discrete Derivative/1
  Product1/1 -> u_4/1, f/1
  [phi] -> Mux3/1
  [psi] -> Mux3/3
  Discrete Derivative2/1 -> Mux4/3
  Discrete Derivative1/1 -> Mux4/2, Product3/2
  J.Rr_dot.Euler_dot/1 -> u_8/1, Subtract2/1
  Subtract1/1 -> J.Rr_dot.Euler_dot/2
  [psi] -> Discrete Derivative2/1
  Product3/1 -> u_6/1, Subtract1/2
  Product2/1 -> u_5/1, Subtract1/1
  f/1 -> Out1/1
  d(T)/d(theta)/1(T) -> u_3/1, Product3/1
  Mux4/1 -> u_7/1, J.Rr_dot.Euler_dot/3
  Subtract2/1 -> u_12/1, Product1/2, Display1/1
  Product/1 -> u_10/1, Display2/1, Product1/1

== system IARC_Nonlinear_Sensors/ARC Controller/Attitutde Control/Subsystem/inv(g) ==
  Constant : Constant  Value=Jx
  Constant1 : Constant  Value=Jy
  Constant2 : Constant  Value=Jyaw
  Constant3 : Constant  Value=0
  Divide : Product  Inputs=*/
  Divide1 : Product  Inputs=**/
  Mux : Mux  Inputs=3
  Mux1 : Mux  Inputs=3
  Mux2 : Mux  Inputs=3
  Trigonometric Function1 : Trigonometry  Operator=cos
  Trigonometric Function2 : Trigonometry  Operator=cos
  inv(g) : Concatenate  NumInputs=3  Mode=Multidimensional array  ConcatenateDimension=2
  Out1 : Outport
  wires:
  [theta] -> Trigonometric Function1/1
  [phi] -> Trigonometric Function2/1
  Constant3/1 -> Mux2/2, Mux2/1, Mux1/3, Mux1/1, Mux/3, Mux/2
  Mux2/1 -> inv(g)/3
  Mux/1 -> inv(g)/1
  inv(g)/1 -> Out1/1
  Trigonometric Function2/1 -> Divide1/2
  Trigonometric Function1/1 -> Divide/2, Divide1/3
  Constant1/1 -> Mux1/2
  Constant2/1 -> Divide1/1
  Constant/1 -> Divide/1
  Divide1/1 -> Mux2/3
  Divide/1 -> Mux/1
  Mux1/1 -> inv(g)/2

== system IARC_Nonlinear_Sensors/ARC Controller/Attitutde Control/Yaw control/Iz . c phi // c theta ==
  Gain1 : Gain  Gain=Ky
  Product2 : Product  Inputs=*//
  cos : Trigonometry  Operator=cos
  cos1 : Trigonometry  Operator=cos
  " " : Outport
  wires:
  Product2/1 -> Gain1/1
  Gain1/1 -> " "/1
  [theta41_est] -> Product2/3
  cos1/1 -> Product2/2
  cos/1 -> Product2/1
  [theta] -> cos1/1
  [phi] -> cos/1

== system IARC_Nonlinear_Sensors/ARC Controller/Attitutde Control/Yaw control/Phi3 ==
  Constant : Constant
  Mux1 : Mux  Inputs=2
  Product2 : Product  Inputs=*/*/
  alpha 42 dot : Subsystem
  cos : Trigonometry
  cos1 : Trigonometry  Operator=cos
  Out1 : Outport
  wires:
  [theta41_est] -> Product2/4
  alpha 42 dot/1(alpha_42_dot) -> Product2/3
  Constant/1 -> Mux1/2
  Product2/1 -> Mux1/1
  Mux1/1 -> Out1/1
  [theta] -> cos/1
  cos/1 -> Product2/1
  [phi] -> cos1/1
  cos1/1 -> Product2/2

== system IARC_Nonlinear_Sensors/ARC Controller/Attitutde Control/Yaw control/Robust term ==
  e : Inport
  phi : Inport  Port=2
  Add : Sum
  Constant3 : Constant  Value=theta_max-theta_min
  Constant6 : Constant  Value=delta
  Gain : Gain  Gain=1/(4*epsilon)
  Math Function : Math  Operator=magnitude^2  SaturateOnIntegerOverflow=on
  Math Function1 : Math  Operator=magnitude^2  SaturateOnIntegerOverflow=on
  Math Function3 : Math  Operator=magnitude^2  SaturateOnIntegerOverflow=on
  Math Function5 : Math  Operator=transpose  SaturateOnIntegerOverflow=on
  Product : Product  Multiplication=Matrix(*)
  Product1 : Product
  alpha : Outport
  wires:
  Gain/1 -> Product1/2
  Add/1 -> Product1/1
  Math Function/1 -> Product/2
  Constant6/1 -> Math Function3/1
  Math Function3/1 -> Add/2
  Product/1 -> Add/1
  Math Function1/1 -> Math Function5/1
  Constant3/1 -> Math Function/1
  Product1/1 -> alpha/1
  Math Function5/1 -> Product/1
  e/1 -> Gain/1
  phi/1 -> Math Function1/1

== system IARC_Nonlinear_Sensors/ARC Controller/Attitutde Control/Yaw control/Subsystem ==
  Phi_D : Inport
  error : Inport  Port=2
  f(x) : Inport  Port=3
  Phi_I : Inport  Port=4
  Adapt : Inport  Port=5
  " " : Subsystem
  Constant1 : Constant  Value=theta4_Min(1,2)
  Constant2 : Constant  Value=theta4_Max(1,2)
  Constant6 : Constant  Value=theta4_Max(1,1)
  Constant7 : Constant  Value=theta4_Min(1,1)
  Demux : Demux  Outputs=2
  Demux1 : Demux  Outputs=2
  Gain1 : Gain
  Gain3 : Gain  Gain=Ky
  "IARC, Physical Model Based Parameter Estimation (69)_Yaw" : Subsystem  AncestorBlock=|  mask(Physical Model Based Parameter Estimation){mu1=mu1_yaw, mu2=mu2_yaw, alpha=alpha3, nu=nu3, gamma0=gamma4_0, Rho_M=Rho_M_yaw, Rho_L=Rho_L_yaw, v=v_yaw, theta_0=theta4_0, theta_max=theta4_Max, theta_min=theta4_Min, Theta_dot_M=theta_dot_M_yaw, Tau=Tau_yaw, t0=t0, Norm_ON=on}
      | UAV_Control/IARC, Physical Model Based 
      | Parameter Estimation (69)
      mask prompts: mu1 "forgetting factor, mu1:"; mu2 "RLS parameter, mu2:"; alpha "forgetting factor, alpha:"; nu "normalizing factor, nu:"; gamma0 "Initial adaptation gain:"; Rho_M "Upper bound for the adaptation gain:"; Rho_L "Lower bound for the adaptation gain:"; v "Eigenvector of Gamma_max:"; Theta_dot_M "Theta dot max:"; Tau "Filter time constant:"; t0 "Initialization Delay:"; Norm_ON "Use Normalized formula"
      mask Help:
      | Filtered system dynamics:
      | H_f (s)  is any stable LTI filter transfer function
      | x_f=H_f [x]
      | φ_f=H_f [φ(x)]
      | u_f=H_f [u]
      | 
      | y_p=x ̇_f−u_f
      | y ̂_p=φ_f^T θ ̂
      | Prediction error:
      | ϵ=y_p−y ̂_p
      | 
      | recursive estimation algorithms, the generalized parameter estimation algorithm (PAA) with covariance limiting:
      | 
      | θ ̂  ̇(t)=Γ(t) φ_f (t)ϵ(t)
      | D_Γ=μ_1 (t)Γ(t)−μ_2 (t)Γ(t) φ_f (t) φ_f (t)^T Γ(t)
      | Γ ̇(t)=D_Γ, if λ_M (Γ(t))<ρ_M  or v_M^T D_Γ v_M<0 )
      |          0        else
      | 
      | μ_1  and μ_2  are two non-negative functions
      | ρ_M  is a preset upper bound for the covariance matrix Γ(t)
      | μ_1  represents the forgetting factor (μ_1=0 for not forgetting)
      | μ_2: 1 stands for the standard least squares type estimation algorithm
      |        0 stands for  the gradient type estimation algorithm
      |        range: 0≤μ_2<2
      | Initialization of the covariance matrix: Γ(0)<ρ_M I_p
      | 
      | IARC designs completely separate the parameter estimation law design from the underlying robust control law to give better parameter estimates than possible with DARC designs. In addition, explicit on-line signal excitation level monitoring can be employed to significantly improve the accuracy of  parameter estimates.
      | 
      | Normalized Method:
      | θ ̂  ̇(t)=(Γ(t) φ_f (t)ϵ(t))/(1+νφ_f^T Γφ_f )
      | D_Γ=αΓ(t)−(Γ(t) φ_f (t) φ_f (t)^T Γ(t))/(1+νφ_f^T Γφ_f )
      | Γ ̇(t)=D_Γ, if λ_M (Γ(t))<ρ_M  or v_M^T D_Γ v_M<0
      |           0       else
      mask Display:
      | port_label('input',1,'f(x)','texmode','on')
      | port_label('input',2,'\phi','texmode','on')
      | port_label('input',3,'Adapt','texmode','on')
      | 
      | port_label('output',1,'\theta_{hat}','texmode','on')
  Integral Type Adaptation Law Discontinuous Projection1 : Subsystem  AncestorBlock=|  mask(IntegralTypeAdaptationLaw){theta=theta4, theta0=theta4_0, theta_max=theta4_Max, theta_min=theta4_Min, gamma=Gamma4, t0=t0, Adaptation_ON=on}
      | UAV_Control/Integral Type
      | Adaptation Law
      | Discontinuous Projection
      mask prompts: theta "Actual value of theta:"; theta0 "Initial value of theta:"; theta_max "Maximum value of theta:"; theta_min "Minimum value of theta:"; gamma "Adaptation Rate:"; t0 "Initialization Delay:"; Adaptation_ON "Activate adaptation:"
      mask help: Applies an Integral-type adaptation law with discontinuous projection on the parameter theta.
      mask Help:
      | Applies an Integral-type adaptation law with discontinuous projection on the parameter theta.
      | 
      | theta_est_dot=Gamma*Phi*e
      | theta=proj( int(theta_estdot) )
      | 
      | theta_min < theta_est <  theta_max
      | 
      | Parameters:
      | 
      | Gamma: nxn diagonal matrix, adaptaion rate.
      | theta_min: nx1 vector, minimum value of the estimated vector.
      | theta_max: nx1 vector, maximum value of the estimated vector.
      | theta0: nx1 vector, initial value of the estimated vector.
      | theta: nx1 vector, actual value of the estimated vector.
      | Adaptation_On: controls the use of the adaptation law (1: active, 0: inactive)
      | 
      | Inputs:
      | Phi: regressor vector, theta0, nx1.
      | e: state error, scalar.
      | 
      | Outputs:
      | theta_est: estimated value of the parameters vector.
      mask Display:
      | port_label('input',1,'\phi','texmode','on')
      | port_label('input',2,'e','texmode','on')
      | port_label('output',1,'\theta_{hat}','texmode','on')
  J : Subsystem
  Jzz : Scope
  Manual Switch : ManualSwitch  CurrentSetting=0
  Manual Switch1 : ManualSwitch  CurrentSetting=0
  Math Function : Math  Operator=reciprocal  SaturateOnIntegerOverflow=on
  Mux3 : Mux  Inputs=5
  Mux6 : Mux  Inputs=5
  Subsystem1 : Subsystem
  To File : ToFile  Commented=on  Filename=IARC41.mat  MatrixName=IARC41  SaveFormat=Timeseries
  To File1 : ToFile  Commented=on  Filename=IARC42.mat  MatrixName=IARC42  SaveFormat=Timeseries
  d4 (N.m) : Scope
  theta1 : Outport
  theta2 : Outport  Port=2
  wires:
  Math Function/1 -> Gain3/1
  Gain3/1 -> To File/1, Jzz/1
  Demux/1 -> Manual Switch/1, Mux3/1
  Mux3/1 -> Math Function/1
  J/1(Out1) -> Mux3/3
  Demux1/1 -> Mux3/2, Manual Switch/2  "Ky/Iz"
  Constant6/1 -> Mux3/4
  Constant7/1 -> Mux3/5
  Integral Type Adaptation Law Discontinuous Projection1/1(theta_est) -> Demux/1
  Phi_D/1 -> Integral Type Adaptation Law Discontinuous Projection1/1(Phi)
  error/1 -> Integral Type Adaptation Law Discontinuous Projection1/2(error)
  Manual Switch/1 -> theta1/1
  Phi_I/1 -> "IARC, Physical Model Based Parameter Estimation (69)_Yaw"/2(Phi)
  f(x)/1 -> "IARC, Physical Model Based Parameter Estimation (69)_Yaw"/1(f(x))
  Adapt/1 -> "IARC, Physical Model Based Parameter Estimation (69)_Yaw"/3(Adapt)
  Subsystem1/1(y) -> To File1/1, d4 (N.m)/1
  Constant2/1 -> Mux6/4
  Demux/2 -> Manual Switch1/1, Mux6/1
  " "/1(Out1) -> Mux6/3  "True"
  Constant1/1 -> Mux6/5
  Mux6/1 -> Subsystem1/1(u)
  Demux1/2 -> Manual Switch1/2, Mux6/2
  Manual Switch1/1 -> Gain1/1
  "IARC, Physical Model Based Parameter Estimation (69)_Yaw"/1(Theta_hat) -> Demux1/1
  Gain1/1 -> theta2/1

== system IARC_Nonlinear_Sensors/ARC Controller/Attitutde Control/Yaw control/T1 .. ==
  "  " : Trigonometry  Operator=cos
  "    " : Trigonometry
  Constant : Constant  Value=Jx
  Gain1 : Gain  Gain=-1
  Product1 : Product  Inputs=*/*/
  Out1 : Outport
  wires:
  Product1/1 -> Gain1/1
  Gain1/1 -> Out1/1
  [T1] -> Product1/3
  Constant/1 -> Product1/4
  [phi] -> "  "/1
  [theta] -> "    "/1
  "    "/1 -> Product1/1
  "  "/1 -> Product1/2
